simulink model "LQRstatespace"  (R2023b)
settings: Solver=ode14x  StartTime=0.0  StopTime=10.0  FixedStep=0.01  RelTol=1e-3
undefined symbols (not defined in the file): A, B, C, D, K_opt
settings Model: Creator=lxy18  LastModifiedBy=lxy18

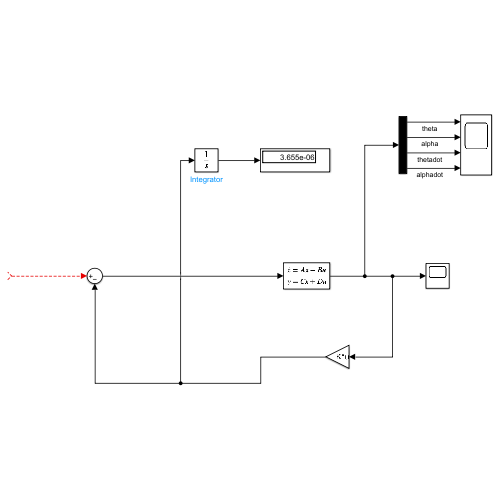
[thumbnail: Simulink's stored preview of the top-level diagram]
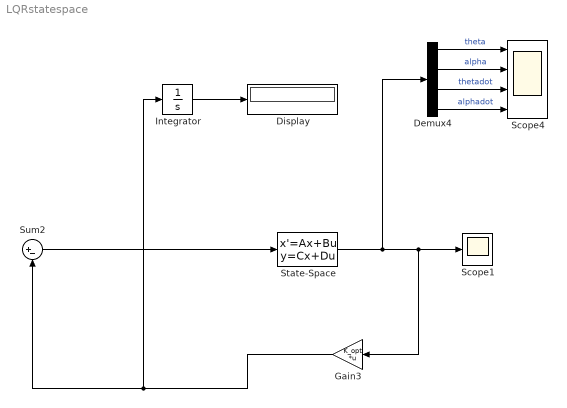
== system LQRstatespace ==
  Demux4 : Demux
  Display : Display
  Gain3 : Gain  Gain=K_opt  Multiplication=Matrix(K*u)
  Integrator : Integrator
  Scope1 : Scope
  Scope4 : Scope  NumInputPorts=4
  State-Space : StateSpace  A=A  B=B  C=C  D=D  InitialCondition=[1 * pi / 180; 1 * pi / 180; 0; 0]
  Sum2 : Sum  Inputs=|+-
  wires:
  State-Space/1 -> Gain3/1, Scope1/1, Demux4/1
  Gain3/1 -> Integrator/1, Sum2/2
  Sum2/1 -> State-Space/1
  Demux4/3 -> Scope4/3  "thetadot"
  Demux4/2 -> Scope4/2  "alpha"
  Demux4/4 -> Scope4/4  "alphadot"
  Demux4/1 -> Scope4/1  "theta"
  ? -> Sum2/1
  Integrator/1 -> Display/1
